simulink model "task10_lab14"  (R2021a)
settings: Solver=FixedStepAuto  StartTime=0.0  StopTime=10.0  FixedStep=0.1  RelTol=1e-3
settings Model: Creator=reemb  LastModifiedBy=reemb

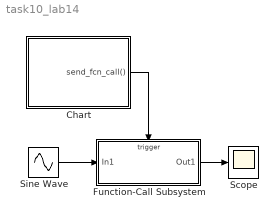
== system task10_lab14 ==
  Chart : Stateflow chart  TreatAsAtomicUnit=on  SystemSampleTime=1
  Function-Call Subsystem : Subsystem  TreatAsAtomicUnit=on
  Scope : Scope
  Sine Wave : Sin  SampleTime=0
  wires:
  Chart/1(send_fcn_call()) -> Function-Call Subsystem/Trigger
  Function-Call Subsystem/1(Out1) -> Scope/1
  Sine Wave/1 -> Function-Call Subsystem/1(In1)

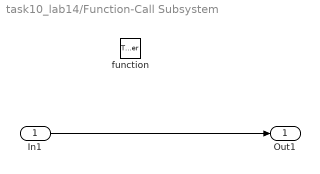
== system task10_lab14/Function-Call Subsystem ==
  In1 : Inport
  function : TriggerPort  TriggerType=function-call  VariantControl=(inherit)
  Out1 : Outport
  wires:
  In1/1 -> Out1/1

== stateflow chart task10_lab14/Chart ==
  state Enabled
    on every(1, tick):
    send_fcn_call();
  state Disabled
  Disabled -> Enabled : (after(3, tick))
  (default) -> Enabled
  Enabled -> Disabled : (after(3, tick))
  events: send_fcn_call output FUNCTION_CALL_EVENT
